simulink model "var30"  (R2020a)
settings: Solver=VariableStepAuto  StartTime=0.0  StopTime=8  RelTol=1e-3
libraries: commseqgen3 x3
settings Model: Creator=User  LastModifiedBy=User

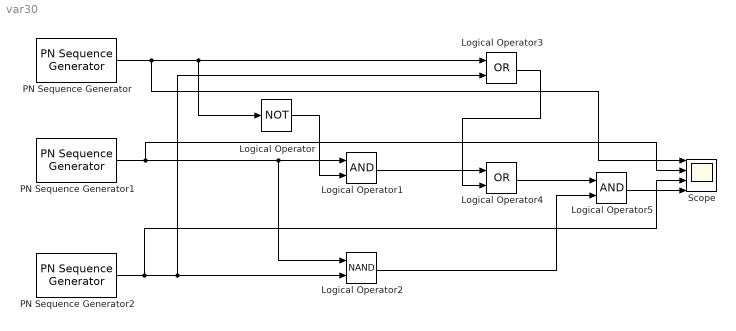
== system var30 ==
  Logical Operator : Logic  Operator=NOT  AllPortsSameDT=off  OutDataTypeStr=boolean
  Logical Operator1 : Logic  AllPortsSameDT=off  OutDataTypeStr=boolean
  Logical Operator2 : Logic  Operator=NAND  AllPortsSameDT=off  OutDataTypeStr=boolean
  Logical Operator3 : Logic  Operator=OR  AllPortsSameDT=off  OutDataTypeStr=boolean
  Logical Operator4 : Logic  Operator=OR  AllPortsSameDT=off  OutDataTypeStr=boolean
  Logical Operator5 : Logic  AllPortsSameDT=off  OutDataTypeStr=boolean
  PN Sequence Generator : commseqgen3/PN Sequence Generator  poly='z^8 + z + 1'  ini_sta=[1 1 1 1 0 0 0 0]  outBitMaskSource=Dialog parameter  shift=0  outVarSiz=off  maxOutSizeMode=Dialog parameter  maxOutSize=[10 1]  Ts=1  sampPerFrame=1  reset=off  bitPackedOutputs=off  outDataType=double  numPackedBits=8  bitPackDataSigned=off  bitPackedOutDType=double
  PN Sequence Generator1 : commseqgen3/PN Sequence Generator  poly='z^8 + z + 1'  ini_sta=[1 1 0 0 1 1 0 0]  outBitMaskSource=Dialog parameter  shift=0  outVarSiz=off  maxOutSizeMode=Dialog parameter  maxOutSize=[10 1]  Ts=1  sampPerFrame=1  reset=off  bitPackedOutputs=off  outDataType=double  numPackedBits=8  bitPackDataSigned=off  bitPackedOutDType=double
  PN Sequence Generator2 : commseqgen3/PN Sequence Generator  poly='z^8 + z + 1'  ini_sta=[1 0 1 0 1 0 1 0]  outBitMaskSource=Dialog parameter  shift=0  outVarSiz=off  maxOutSizeMode=Dialog parameter  maxOutSize=[10 1]  Ts=1  sampPerFrame=1  reset=off  bitPackedOutputs=off  outDataType=double  numPackedBits=8  bitPackDataSigned=off  bitPackedOutDType=double
  Scope : Scope  NumInputPorts=4
  wires:
  PN Sequence Generator/1 -> Scope/1, Logical Operator/1, Logical Operator3/1
  PN Sequence Generator1/1 -> Scope/2, Logical Operator2/1, Logical Operator1/1
  Logical Operator/1 -> Logical Operator1/2
  PN Sequence Generator2/1 -> Scope/3, Logical Operator3/2, Logical Operator2/2
  Logical Operator1/1 -> Logical Operator4/1
  Logical Operator3/1 -> Logical Operator4/2
  Logical Operator4/1 -> Logical Operator5/1
  Logical Operator2/1 -> Logical Operator5/2
  Logical Operator5/1 -> Scope/4
